simulink model "QuadRotorPlant"  (R2014b)
settings: Solver=ode23t  StartTime=0.0  StopTime=15  RelTol=1e-3
undefined symbols (not defined in the file): Ap, getArbitraryAngle, getArbitraryAxis, kt, L, Pitch_0, rho, Roll_0, Rp, X, Y, Z, zInit
libraries: sm_lib x125, fl_lib x106, nesl_utility x49, elec_lib x12, aerolibtransform2 x4, aerolibconvert2 x2
(part 1 of 4)
settings Model: Creator=ppreethi  LastModifiedBy=syoon
settings DataIOCC: SaveOutput=off  SaveTime=off
settings DebuggingCC: UnderspecifiedInitializationDetection=Classic  MergeDetectMultiDrivingBlocksExec=none  StateNameClashWarn=warning
settings SimscapeCC: SelectedTab=SimMechanics2G

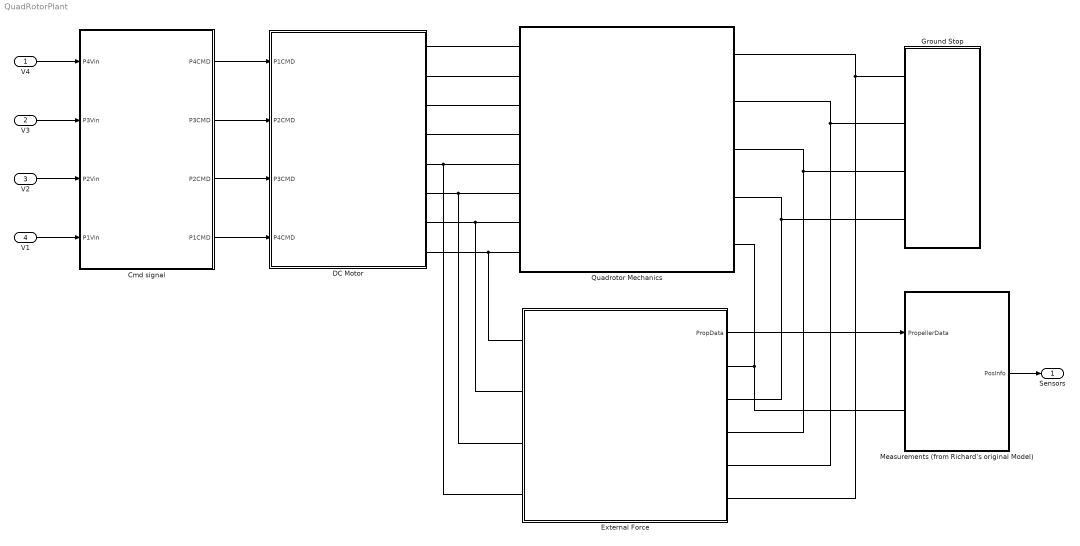
== system QuadRotorPlant ==
  V4 : Inport  OutDataTypeStr=double  PortDimensions=1  SampleTime=[0.01,0]
  V3 : Inport  Port=2  OutDataTypeStr=double  PortDimensions=1  SampleTime=[0.01,0]
  V2 : Inport  Port=3  OutDataTypeStr=double  PortDimensions=1  SampleTime=[0.01,0]
  V1 : Inport  Port=4  OutDataTypeStr=double  PortDimensions=1  SampleTime=[0.01,0]
  Cmd signal : Subsystem
  DC Motor : Subsystem
      mask Display: image(imread('motor.jpg'))
  External Force : Subsystem
  Ground Stop : Subsystem  mask{Roll0=Roll_0, Pitch0=Pitch_0, Yaw0=0, Damp=0.7, Spring=1e2, Length=-0.083057999999999979068, GRoll=0, GPitch=0, Alt=0}
      mask prompts: Roll0 "Init Roll"; Pitch0 "Init Pitch"; Yaw0 "Init Yaw"; Damp "Damping"; Spring "Spring Constant"; Length "Distance from Center to Motor"; GRoll "Ground Roll"; GPitch "Ground Pitch"; Alt "Initial Altitude"
      mask init:
      | blk = gcb;
      | if Alt<0
      |     Alt = 0;
      |     set_param(blk,'Alt','0')
      |     warning('Cannot Initialize Below Zero Altitude');
      | end
  Measurements (from Richard's original Model) : Subsystem
  Quadrotor Mechanics : Subsystem
  Sensors : Outport  OutDataTypeStr=Bus: VehicleStates  PortDimensions=1  SampleTime=0  BusOutputAsStruct=on
  wires:
  Cmd signal/1(P4CMD) -> DC Motor/1(P1CMD)
  Cmd signal/2(P3CMD) -> DC Motor/2(P2CMD)
  Cmd signal/3(P2CMD) -> DC Motor/3(P3CMD)
  Cmd signal/4(P1CMD) -> DC Motor/4(P4CMD)
  Measurements (from Richard's original Model)/1(PosInfo) -> Sensors/1
  V2/1 -> Cmd signal/3(P2Vin)
  V3/1 -> Cmd signal/2(P3Vin)
  V1/1 -> Cmd signal/4(P1Vin)
  V4/1 -> Cmd signal/1(P4Vin)
  External Force/1(PropData) -> Measurements (from Richard's original Model)/1(PropellerData)
  connections:
  Quadrotor Mechanics/LConn8 -- External Force/LConn1 -- DC Motor/RConn8
  External Force/LConn2 -- Quadrotor Mechanics/LConn7 -- DC Motor/RConn7
  External Force/LConn4 -- DC Motor/RConn5 -- Quadrotor Mechanics/LConn5
  Ground Stop/RConn1 -- External Force/RConn5 -- Quadrotor Mechanics/RConn1
  Ground Stop/RConn3 -- External Force/RConn3 -- Quadrotor Mechanics/RConn3
  Ground Stop/RConn2 -- External Force/RConn4 -- Quadrotor Mechanics/RConn2
  Ground Stop/RConn4 -- External Force/RConn2 -- Quadrotor Mechanics/RConn4
  External Force/RConn1 -- Measurements (from Richard's original Model)/LConn1 -- Quadrotor Mechanics/RConn5
  Quadrotor Mechanics/LConn6 -- External Force/LConn3 -- DC Motor/RConn6
  DC Motor/RConn4 -- Quadrotor Mechanics/LConn4
  DC Motor/RConn3 -- Quadrotor Mechanics/LConn3
  DC Motor/RConn2 -- Quadrotor Mechanics/LConn2
  DC Motor/RConn1 -- Quadrotor Mechanics/LConn1

== system QuadRotorPlant/Cmd signal ==
  P4Vin : Inport
  P3Vin : Inport  Port=2
  P2Vin : Inport  Port=3
  P1Vin : Inport  Port=4
  Bus Creator{1..4} (4 alike) : BusCreator  Inputs=2
  CMD : Subsystem
  CMD1 : Subsystem
  CMD2 : Subsystem
  CMD3 : Subsystem
  P4CMD : Outport
  P3CMD : Outport  Port=2
  P2CMD : Outport  Port=3
  P1CMD : Outport  Port=4
  wires:
  CMD3/2(REV) -> Bus Creator3/2  "rev"
  CMD3/1(Duty) -> Bus Creator3/1  "duty"
  CMD2/2(REV) -> Bus Creator2/2  "rev"
  CMD2/1(Duty) -> Bus Creator2/1  "duty"
  CMD1/2(REV) -> Bus Creator1/2  "rev"
  CMD1/1(Duty) -> Bus Creator1/1  "duty"
  Bus Creator1/1 -> P3CMD/1  "P2CMD"
  Bus Creator3/1 -> P1CMD/1  "P4CMD"
  Bus Creator2/1 -> P2CMD/1  "P3CMD"
  CMD/2(REV) -> Bus Creator4/2  "rev"
  CMD/1(Duty) -> Bus Creator4/1  "duty"
  Bus Creator4/1 -> P4CMD/1  "P1CMD"
  P3Vin/1 -> CMD1/1(Vcmd)
  P1Vin/1 -> CMD3/1(Vcmd)
  P2Vin/1 -> CMD2/1(Vcmd)
  P4Vin/1 -> CMD/1(Vcmd)

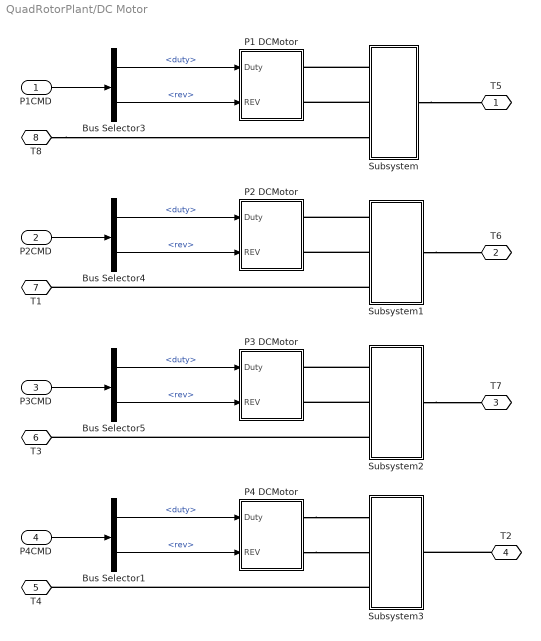
== system QuadRotorPlant/DC Motor ==
  P1CMD : Inport
  P2CMD : Inport  Port=2
  P3CMD : Inport  Port=3
  P4CMD : Inport  Port=4
  Bus Selector{1,3..5} (4 alike) : BusSelector  OutputSignals=duty,rev
  P1 DCMotor : Subsystem
      mask Display: image(imread('motor.jpg'))
  P2 DCMotor : Subsystem
      mask Display: image(imread('motor.jpg'))
  P3 DCMotor : Subsystem
      mask Display: image(imread('motor.jpg'))
  P4 DCMotor : Subsystem
      mask Display: image(imread('motor.jpg'))
  Subsystem : Subsystem
  Subsystem1 : Subsystem
  Subsystem2 : Subsystem
  Subsystem3 : Subsystem
  T5 : PMIOPort  Port=1  Side=Right
  T6 : PMIOPort  Port=2  Side=Right
  T7 : PMIOPort  Port=3  Side=Right
  T2 : PMIOPort  Port=4  Side=Right
  T4 : PMIOPort  Port=5  Side=Right
  T3 : PMIOPort  Port=6  Side=Right
  T1 : PMIOPort  Port=7  Side=Right
  T8 : PMIOPort  Port=8  Side=Right
  wires:
  Bus Selector1/1 -> P4 DCMotor/1(Duty)  "<duty>"
  Bus Selector1/2 -> P4 DCMotor/2(REV)  "<rev>"
  Bus Selector5/1 -> P3 DCMotor/1(Duty)  "<duty>"
  Bus Selector5/2 -> P3 DCMotor/2(REV)  "<rev>"
  Bus Selector4/1 -> P2 DCMotor/1(Duty)  "<duty>"
  Bus Selector4/2 -> P2 DCMotor/2(REV)  "<rev>"
  P2CMD/1 -> Bus Selector4/1
  P4CMD/1 -> Bus Selector1/1
  P3CMD/1 -> Bus Selector5/1
  P1CMD/1 -> Bus Selector3/1
  Bus Selector3/1 -> P1 DCMotor/1(Duty)  "<duty>"
  Bus Selector3/2 -> P1 DCMotor/2(REV)  "<rev>"
  connections:
  T8/RConn1 -- Subsystem/LConn3
  Subsystem1/LConn3 -- T1/RConn1
  Subsystem2/LConn3 -- T3/RConn1
  Subsystem3/LConn3 -- T4/RConn1
  T2/RConn1 -- Subsystem3/RConn1
  Subsystem2/RConn1 -- T7/RConn1
  Subsystem1/RConn1 -- T6/RConn1
  Subsystem/RConn1 -- T5/RConn1
  P4 DCMotor/RConn2 -- Subsystem3/LConn2
  P4 DCMotor/RConn1 -- Subsystem3/LConn1
  Subsystem2/LConn1 -- P3 DCMotor/RConn1
  Subsystem2/LConn2 -- P3 DCMotor/RConn2
  Subsystem1/LConn1 -- P2 DCMotor/RConn1
  Subsystem1/LConn2 -- P2 DCMotor/RConn2
  Subsystem/LConn2 -- P1 DCMotor/RConn2
  Subsystem/LConn1 -- P1 DCMotor/RConn1

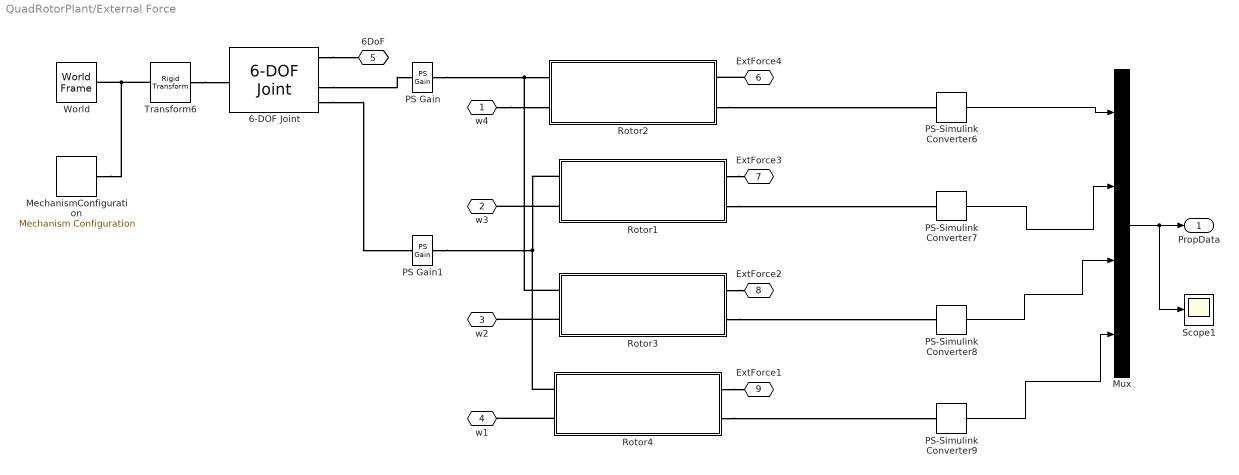
== system QuadRotorPlant/External Force ==
  6-DOF Joint : sm_lib/Joints/6-DOF Joint  SenseConstraintForce=off  SenseConstraintForceX=off  SenseConstraintForceY=off  SenseConstraintForceZ=off  SenseConstraintTorque=off  SenseConstraintTorqueX=off  SenseConstraintTorqueY=off  SenseConstraintTorqueZ=off  SenseTotalForce=off  SenseTotalForceX=off  SenseTotalForceY=off  SenseTotalForceZ=off  SenseTotalTorque=off  SenseTotalTorqueX=off  SenseTotalTorqueY=off  SenseTotalTorqueZ=off  CompositeWrenchDir=FollowerOnBase  CompositeWrenchFrame=BaseFrame  PxEquilibriumPosition=0  PxEquilibriumPositionUnits=m  PxSpringStiffness=0  PxSpringStiffnessUnits=N/m  PxDampingCoefficient=0  PxDampingCoefficientUnits=N/(m/s)  PxTorqueActuationMode=NoTorque  PxMotionActuationMode=ComputedMotion  PxSensePosition=off  PxSenseVelocity=off  PxSenseAcceleration=off  PxSenseTorqueForce=off  PxPositionTargetValue=0  PxPositionTargetValueUnits=m  PxPositionTargetSpecify=off  PxPositionTargetPriority=High  PxVelocityTargetValue=0  PxVelocityTargetValueUnits=m/s  PxVelocityTargetSpecify=off  PxVelocityTargetPriority=High  PyEquilibriumPosition=0  PyEquilibriumPositionUnits=m  PySpringStiffness=0  PySpringStiffnessUnits=N/m  PyDampingCoefficient=0  PyDampingCoefficientUnits=N/(m/s)  PyTorqueActuationMode=NoTorque  PyMotionActuationMode=ComputedMotion  PySensePosition=off  PySenseVelocity=off  PySenseAcceleration=off  PySenseTorqueForce=off  PyPositionTargetValue=0  PyPositionTargetValueUnits=m  PyPositionTargetSpecify=off  PyPositionTargetPriority=High  PyVelocityTargetValue=0  PyVelocityTargetValueUnits=m/s  PyVelocityTargetSpecify=off  PyVelocityTargetPriority=High  PzEquilibriumPosition=0  PzEquilibriumPositionUnits=m  PzSpringStiffness=0  PzSpringStiffnessUnits=N/m  PzDampingCoefficient=0  PzDampingCoefficientUnits=N/(m/s)  PzTorqueActuationMode=NoTorque  PzMotionActuationMode=ComputedMotion  PzSensePosition=off  PzSenseVelocity=on  PzSenseAcceleration=off  PzSenseTorqueForce=off  PzPositionTargetValue=0  PzPositionTargetValueUnits=m  PzPositionTargetSpecify=off  PzPositionTargetPriority=High  PzVelocityTargetValue=0  PzVelocityTargetValueUnits=m/s  PzVelocityTargetSpecify=off  PzVelocityTargetPriority=High  SphDefPosRotationMethod=None  SphDefPosRotationAngleUnits=deg  SphDefPosRotationStandardAxis=+Z  SphDefPosRotationAngle=0  SphDefPosRotationArbitraryAxis=[0 0 1]  SphDefPosFollAlignAxisA=+X  SphDefPosBaseAlignAxisA=+Y  SphDefPosFollAlignAxisB=+Y  SphDefPosBaseAlignAxisB=+Z  SphDefPosRotationMatrix=[1 0 0; 0 1 0; 0 0 1]  SphEqPosRotationMethod=None  SphEqPosRotationAngleUnits=deg  SphEqPosRotationStandardAxis=+Z  SphEqPosRotationAngle=0  SphEqPosRotationArbitraryAxis=[0 0 1]  SphEqPosFollAlignAxisA=+X  SphEqPosBaseAlignAxisA=+Y  SphEqPosFollAlignAxisB=+Y  SphEqPosBaseAlignAxisB=+Z  SphEqPosRotationMatrix=[1 0 0; 0 1 0; 0 0 1]  SphSpringStiffness=0  SphSpringStiffnessUnits=N*m/deg  SphDampingCoefficient=0  SphDampingCoefficientUnits=N*m/(deg/s)  SphActuateTorqueX=off  SphActuateTorqueY=off  SphActuateTorqueZ=off  SphActuateTorque=off  SphTorqueActuationMode=NoTorque  SphMotionActuationMode=ComputedMotion  SphActuationFrame=BaseFrame  SphSensePosition=off  SphSenseVelocityX=on  SphSenseVelocityY=on  SphSenseVelocityZ=off  SphSenseVelocity=off  SphSenseAccelerationX=off  SphSenseAccelerationY=off  SphSenseAccelerationZ=off  SphSenseAcceleration=off  SphSenseTorqueX=off  SphSenseTorqueY=off  SphSenseTorqueZ=off  SphSenseTorqueForce=off  SphSensingFrame=BaseFrame  SphPositionTargetRotationMethod=None  SphPositionTargetRotationAngleUnits=deg  SphPositionTargetRotationStandardAxis=+Z  SphPositionTargetRotationAngle=0  SphPositionTargetRotationArbitraryAxis=[0 0 1]  SphPositionTargetFollAlignAxisA=+X  SphPositionTargetBaseAlignAxisA=+Y  SphPositionTargetFollAlignAxisB=+Y  SphPositionTargetBaseAlignAxisB=+Z  SphPositionTargetRotationMatrix=[1 0 0; 0 1 0; 0 0 1]  SphPositionTargetSpecify=off  SphPositionTargetPriority=High  SphVelocityTargetValue=[0 0 0]  SphVelocityTargetValueUnits=deg/s  SphVelocityTargetSpecify=off  SphVelocityTargetPriority=High  SphVelocityTargetInFollowerFrame=on  BlockFunction=simmechanics.library.joints.sixdof_joint
  MechanismConfiguration : sm_lib/Utilities/Mechanism Configuration  UniformGravity=Constant  GravityVector=[0 0 9.81]  GravityUnits=m/s^2  LinearizationDelta=0.001  BlockFunction=simmechanics.library.utilities.mechanism_configuration
  Mux : Mux
  PS Gain : fl_lib/Physical Signals/Functions/PS Gain  gain=pi/180
  PS Gain1 : fl_lib/Physical Signals/Functions/PS Gain  gain=pi/180
  PS-Simulink Converter{6..9} (4 alike) : nesl_utility/PS-Simulink Converter  PhysicalDomain=network_engine_domain  SubClassName=ps_output  LeftPortType=input  RightPortType=output  PseudoPeriodic=off  Frequencies=[]  Unit=1  AffineConversion=off
  Rotor1 : Subsystem
  Rotor2 : Subsystem
  Rotor3 : Subsystem
  Rotor4 : Subsystem
  Scope1 : Scope
      settings: TimeRange=5  YMin=-0.025  YMax=0.25  SaveName=ScopeData11
  Transform6 : sm_lib/Frames and Transforms/Rigid Transform  TranslationMethod=None  TranslationLengthUnit=m  TranslationStandardAxis=+Z  TranslationStandardOffset=0  TranslationCartesianOffset=[0 0 0]  TranslationROffset=0  TranslationROffsetUnits=m  TranslationZOffset=0  TranslationZOffsetUnits=m  TranslationThetaOffset=0  TranslationThetaOffsetUnits=deg  RotationMethod=StandardAxis  RotationAngleUnits=deg  RotationStandardAxis=+X  RotationAngle=180  RotationArbitraryAxis=[0 0 1]  FollAlignAxisA=+X  BaseAlignAxisA=+Y  FollAlignAxisB=+Y  BaseAlignAxisB=+Z  RotationMatrix=[1 0 0; 0 1 0; 0 0 1]  BlockFunction=simmechanics.library.frames_transforms.rigid_transform
  World : sm_lib/Frames and Transforms/World Frame  BlockFunction=simmechanics.library.frames_transforms.world_frame
  w4 : PMIOPort  Port=1  Side=Left
  w3 : PMIOPort  Port=2  Side=Left
  w2 : PMIOPort  Port=3  Side=Left
  w1 : PMIOPort  Port=4  Side=Left
  6DoF : PMIOPort  Port=5  Side=Right
  ExtForce4 : PMIOPort  Port=6  Side=Right
  ExtForce3 : PMIOPort  Port=7  Side=Right
  ExtForce2 : PMIOPort  Port=8  Side=Right
  ExtForce1 : PMIOPort  Port=9  Side=Right
  PropData : Outport
  wires:
  Mux/1 -> PropData/1, Scope1/1
  PS-Simulink Converter6/1 -> Mux/1
  PS-Simulink Converter7/1 -> Mux/2
  PS-Simulink Converter8/1 -> Mux/3
  PS-Simulink Converter9/1 -> Mux/4
  connections:
  6-DOF Joint/RConn3 -- PS Gain/LConn1
  6-DOF Joint/RConn4 -- PS Gain1/LConn1
  MechanismConfiguration/RConn1 -- World/RConn1 -- Transform6/LConn1
  Transform6/RConn1 -- 6-DOF Joint/LConn1
  6-DOF Joint/RConn1 -- 6DoF/RConn1
  Rotor4/LConn2 -- w1/RConn1
  Rotor3/LConn2 -- w2/RConn1
  w4/RConn1 -- Rotor2/LConn2
  ExtForce4/RConn1 -- Rotor2/RConn1
  Rotor1/RConn1 -- ExtForce3/RConn1
  Rotor2/RConn2 -- PS-Simulink Converter6/LConn1
  PS Gain/RConn1 -- Rotor3/LConn1 -- Rotor2/LConn1
  Rotor3/RConn1 -- ExtForce2/RConn1
  Rotor1/LConn1 -- Rotor4/LConn1 -- PS Gain1/RConn1
  Rotor1/RConn2 -- PS-Simulink Converter7/LConn1
  Rotor1/LConn2 -- w3/RConn1
  Rotor3/RConn2 -- PS-Simulink Converter8/LConn1
  Rotor4/RConn2 -- PS-Simulink Converter9/LConn1
  Rotor4/RConn1 -- ExtForce1/RConn1

== system QuadRotorPlant/Ground Stop ==
  FloorStop1 : Subsystem
  FloorStop2 : Subsystem
  FloorStop3 : Subsystem
  FloorStop4 : Subsystem
  Ground : sm_lib/Body Elements/Solid  InertiaType=CalculateFromGeometry  Mass=1  MassUnits=kg  CenterOfMass=[0 0 0]  CenterOfMassUnits=m  MomentsOfInertia=[1 1 1]  MomentsOfInertiaUnits=kg*m^2  ProductsOfInertia=[0 0 0]  ProductsOfInertiaUnits=kg*m^2  DensityBased=on  Density=2000  DensityUnits=kg/(m^3)  GraphicType=FromGeometry  MarkerShape=Sphere  MarkerSize=10  MarkerSizeUnits=m  GraphicVisPropType=SimpleVisualProperties  GraphicDiffuseColor=[0.0 0.0 0.2]  GraphicSpecularColor=[0.5 0.5 0.5 1.0]  GraphicAmbientColor=[0.15 0.15 0.15 1.0]  GraphicEmissiveColor=[0.0 0.0 0.0 1.0]  GraphicShininess=75  GraphicOpacity=1.0  GeometryShape=Brick  RectangleSize=[1 1]  RectangleSizeUnits=m  BrickDimensions=[1 1 0.01]  BrickDimensionUnits=m  CylinderRadius=1  CylinderRadiusUnits=m  CylinderLength=1  CylinderLengthUnits=m  SphereRadius=1  SphereRadiusUnits=m  EllipsoidRadii=[1 1 1]  EllipsoidRadiiUnits=m  ExtrusionCrossSection=[1 1; -1 1; -1 -1; 1 -1]  ExtrusionCrossSectionUnits=m  ExtrusionLength=1  ExtrusionLengthUnits=m  PolygonNumSides=3  PolygonOuterRadius=1  PolygonOuterRadiusUnits=m  ExtGeomFileType=STL  ExtGeomFileUnits=m  RevolutionCrossSection=[1 1; 1 -1; 2 -1; 2 1]  RevolutionCrossSectionUnits=m  RevolutionExtent=Full  RevolutionAngle=180  RevolutionAngleUnits=deg  BlockFunction=simmechanics.library.body_elements.solid
  Transform1 : sm_lib/Frames and Transforms/Rigid Transform  TranslationMethod=None  TranslationLengthUnit=m  TranslationStandardAxis=+Z  TranslationStandardOffset=0  TranslationCartesianOffset=[0 0 -Alt-0.038]  TranslationROffset=0  TranslationROffsetUnits=m  TranslationZOffset=0  TranslationZOffsetUnits=m  TranslationThetaOffset=0  TranslationThetaOffsetUnits=deg  RotationMethod=ArbitraryAxis  RotationAngleUnits=deg  RotationStandardAxis=+X  RotationAngle=-getArbitraryAngle(GPitch,GRoll,Yaw0)  RotationArbitraryAxis=getArbitraryAxis(GPitch,GRoll,Yaw0);  FollAlignAxisA=-Z  BaseAlignAxisA=+Y  FollAlignAxisB=-Y  BaseAlignAxisB=+X  RotationMatrix=[1 0 0; 0 1 0; 0 0 1]  BlockFunction=simmechanics.library.frames_transforms.rigid_transform
  Transform2 : sm_lib/Frames and Transforms/Rigid Transform  TranslationMethod=Cartesian  TranslationLengthUnit=m  TranslationStandardAxis=+Z  TranslationStandardOffset=0  TranslationCartesianOffset=[0 0 -Alt-0.038]  TranslationROffset=0  TranslationROffsetUnits=m  TranslationZOffset=0  TranslationZOffsetUnits=m  TranslationThetaOffset=0  TranslationThetaOffsetUnits=deg  RotationMethod=StandardAxis  RotationAngleUnits=deg  RotationStandardAxis=+X  RotationAngle=180  RotationArbitraryAxis=getArbitraryAxis(GRoll,GPitch,0);  FollAlignAxisA=-Z  BaseAlignAxisA=+Y  FollAlignAxisB=-Y  BaseAlignAxisB=+X  RotationMatrix=[1 0 0; 0 1 0; 0 0 1]  BlockFunction=simmechanics.library.frames_transforms.rigid_transform
  Transform6 : sm_lib/Frames and Transforms/Rigid Transform  TranslationMethod=None  TranslationLengthUnit=m  TranslationStandardAxis=+Z  TranslationStandardOffset=0  TranslationCartesianOffset=[0 0 0]  TranslationROffset=0  TranslationROffsetUnits=m  TranslationZOffset=0  TranslationZOffsetUnits=m  TranslationThetaOffset=0  TranslationThetaOffsetUnits=deg  RotationMethod=StandardAxis  RotationAngleUnits=deg  RotationStandardAxis=+X  RotationAngle=180  RotationArbitraryAxis=[0 0 1]  FollAlignAxisA=+X  BaseAlignAxisA=+Y  FollAlignAxisB=+Y  BaseAlignAxisB=+Z  RotationMatrix=[1 0 0; 0 1 0; 0 0 1]  BlockFunction=simmechanics.library.frames_transforms.rigid_transform
  World1 : sm_lib/Frames and Transforms/World Frame  BlockFunction=simmechanics.library.frames_transforms.world_frame
  Conn1 : PMIOPort  Port=1  Side=Right
  Conn2 : PMIOPort  Port=2  Side=Right
  Conn3 : PMIOPort  Port=3  Side=Right
  Conn4 : PMIOPort  Port=4  Side=Right
  connections:
  Transform6/LConn1 -- World1/RConn1
  Transform1/RConn1 -- Transform2/LConn1
  Transform1/LConn1 -- Ground/RConn1
  FloorStop1/LConn1 -- FloorStop4/LConn1 -- FloorStop2/LConn1 -- Transform2/RConn1 -- Transform6/RConn1 -- FloorStop3/LConn1
  Conn4/RConn1 -- FloorStop3/RConn1
  Conn2/RConn1 -- FloorStop2/RConn1
  Conn3/RConn1 -- FloorStop1/RConn1
  FloorStop4/RConn1 -- Conn1/RConn1

== system QuadRotorPlant/Measurements (from Richard's original Model) ==
  PropellerData : Inport
  Aerodynamic Drag : Subsystem
  6dof : PMIOPort  Port=1  Side=Left
  PosInfo : Outport  OutDataTypeStr=Bus: VehicleStates
  wires:
  PropellerData/1 -> Aerodynamic Drag/1(PropData)
  Aerodynamic Drag/1(posInfo) -> PosInfo/1
  connections:
  Aerodynamic Drag/LConn1 -- 6dof/RConn1

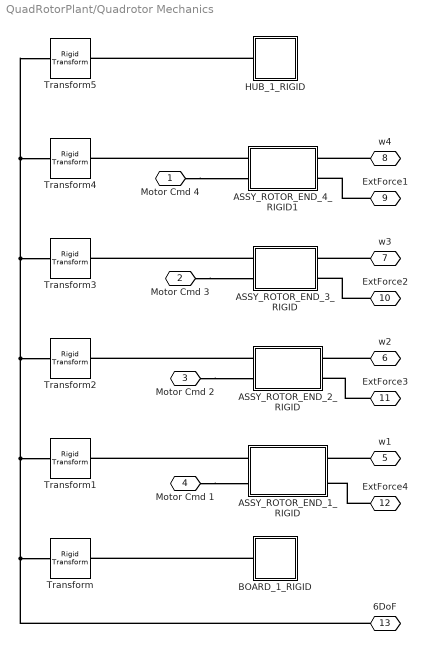
== system QuadRotorPlant/Quadrotor Mechanics ==
  ASSY_ROTOR_END_1_RIGID : Subsystem
  ASSY_ROTOR_END_2_RIGID : Subsystem
  ASSY_ROTOR_END_3_RIGID : Subsystem
  ASSY_ROTOR_END_4_RIGID1 : Subsystem
  BOARD_1_RIGID : Subsystem
  HUB_1_RIGID : Subsystem
  Transform : sm_lib/Frames and Transforms/Rigid Transform  TranslationMethod=Cartesian  TranslationLengthUnit=in  TranslationStandardAxis=+Z  TranslationStandardOffset=0  TranslationCartesianOffset=[0 0 0.27699999999999997]  TranslationROffset=0  TranslationROffsetUnits=m  TranslationZOffset=0  TranslationZOffsetUnits=m  TranslationThetaOffset=0  TranslationThetaOffsetUnits=deg  RotationMethod=ArbitraryAxis  RotationAngleUnits=rad  RotationStandardAxis=+Z  RotationAngle=2.3561943620144121  RotationArbitraryAxis=[-0 -0 -0.99999999999999989]  FollAlignAxisA=+X  BaseAlignAxisA=+Y  FollAlignAxisB=+Y  BaseAlignAxisB=+Z  RotationMatrix=[1 0 0; 0 1 0; 0 0 1]  BlockFunction=simmechanics.library.frames_transforms.rigid_transform
  Transform1 : sm_lib/Frames and Transforms/Rigid Transform  TranslationMethod=Cartesian  TranslationLengthUnit=in  TranslationStandardAxis=+Z  TranslationStandardOffset=0  TranslationCartesianOffset=[0.085999999999999979 -5.5118110236220464e-05 5.5118110236220464e-05]  TranslationROffset=0  TranslationROffsetUnits=m  TranslationZOffset=0  TranslationZOffsetUnits=m  TranslationThetaOffset=0  TranslationThetaOffsetUnits=deg  RotationMethod=None  RotationAngleUnits=deg  RotationStandardAxis=+Z  RotationAngle=0  RotationArbitraryAxis=[0 0 1]  FollAlignAxisA=+X  BaseAlignAxisA=+Y  FollAlignAxisB=+Y  BaseAlignAxisB=+Z  RotationMatrix=[1 0 0; 0 1 0; 0 0 1]  BlockFunction=simmechanics.library.frames_transforms.rigid_transform
  Transform2 : sm_lib/Frames and Transforms/Rigid Transform  TranslationMethod=Cartesian  TranslationLengthUnit=in  TranslationStandardAxis=+Z  TranslationStandardOffset=0  TranslationCartesianOffset=[-5.5118110236220464e-05 -0.085999999999999979 5.5118110236220464e-05]  TranslationROffset=0  TranslationROffsetUnits=m  TranslationZOffset=0  TranslationZOffsetUnits=m  TranslationThetaOffset=0  TranslationThetaOffsetUnits=deg  RotationMethod=ArbitraryAxis  RotationAngleUnits=rad  RotationStandardAxis=+Z  RotationAngle=1.5707963267948968  RotationArbitraryAxis=[-0 -0 -1]  FollAlignAxisA=+X  BaseAlignAxisA=+Y  FollAlignAxisB=+Y  BaseAlignAxisB=+Z  RotationMatrix=[1 0 0; 0 1 0; 0 0 1]  BlockFunction=simmechanics.library.frames_transforms.rigid_transform
  Transform3 : sm_lib/Frames and Transforms/Rigid Transform  TranslationMethod=Cartesian  TranslationLengthUnit=in  TranslationStandardAxis=+Z  TranslationStandardOffset=0  TranslationCartesianOffset=[-0.085999999999999979 5.5118110236220464e-05 5.5118110236220464e-05]  TranslationROffset=0  TranslationROffsetUnits=m  TranslationZOffset=0  TranslationZOffsetUnits=m  TranslationThetaOffset=0  TranslationThetaOffsetUnits=deg  RotationMethod=ArbitraryAxis  RotationAngleUnits=rad  RotationStandardAxis=+Z  RotationAngle=3.1415926535897931  RotationArbitraryAxis=[0 0 1]  FollAlignAxisA=+X  BaseAlignAxisA=+Y  FollAlignAxisB=+Y  BaseAlignAxisB=+Z  RotationMatrix=[1 0 0; 0 1 0; 0 0 1]  BlockFunction=simmechanics.library.frames_transforms.rigid_transform
  Transform4 : sm_lib/Frames and Transforms/Rigid Transform  TranslationMethod=Cartesian  TranslationLengthUnit=in  TranslationStandardAxis=+Z  TranslationStandardOffset=0  TranslationCartesianOffset=[5.5118110236220464e-05 0.085999999999999979 5.5118110236220464e-05]  TranslationROffset=0  TranslationROffsetUnits=m  TranslationZOffset=0  TranslationZOffsetUnits=m  TranslationThetaOffset=0  TranslationThetaOffsetUnits=deg  RotationMethod=ArbitraryAxis  RotationAngleUnits=rad  RotationStandardAxis=+Z  RotationAngle=1.5707963267948968  RotationArbitraryAxis=[0 0 1]  FollAlignAxisA=+X  BaseAlignAxisA=+Y  FollAlignAxisB=+Y  BaseAlignAxisB=+Z  RotationMatrix=[1 0 0; 0 1 0; 0 0 1]  BlockFunction=simmechanics.library.frames_transforms.rigid_transform
  Transform5 : sm_lib/Frames and Transforms/Rigid Transform  TranslationMethod=None  TranslationLengthUnit=m  TranslationStandardAxis=+Z  TranslationStandardOffset=0  TranslationCartesianOffset=[0 0 0]  TranslationROffset=0  TranslationROffsetUnits=m  TranslationZOffset=0  TranslationZOffsetUnits=m  TranslationThetaOffset=0  TranslationThetaOffsetUnits=deg  RotationMethod=None  RotationAngleUnits=deg  RotationStandardAxis=+Z  RotationAngle=0  RotationArbitraryAxis=[0 0 1]  FollAlignAxisA=+X  BaseAlignAxisA=+Y  FollAlignAxisB=+Y  BaseAlignAxisB=+Z  RotationMatrix=[1 0 0; 0 1 0; 0 0 1]  BlockFunction=simmechanics.library.frames_transforms.rigid_transform
  Motor Cmd 4 : PMIOPort  Port=1  Side=Left
  Motor Cmd 3 : PMIOPort  Port=2  Side=Left
  Motor Cmd 2 : PMIOPort  Port=3  Side=Left
  Motor Cmd 1 : PMIOPort  Port=4  Side=Left
  w1 : PMIOPort  Port=5  Side=Left
  w2 : PMIOPort  Port=6  Side=Left
  w3 : PMIOPort  Port=7  Side=Left
  w4 : PMIOPort  Port=8  Side=Left
  ExtForce1 : PMIOPort  Port=9  Side=Right
  ExtForce2 : PMIOPort  Port=10  Side=Right
  ExtForce3 : PMIOPort  Port=11  Side=Right
  ExtForce4 : PMIOPort  Port=12  Side=Right
  6DoF : PMIOPort  Port=13  Side=Right
  connections:
  ASSY_ROTOR_END_4_RIGID1/LConn1 -- Transform4/RConn1
  ASSY_ROTOR_END_2_RIGID/LConn1 -- Transform2/RConn1
  6DoF/RConn1 -- Transform1/LConn1 -- Transform2/LConn1 -- Transform3/LConn1 -- Transform5/LConn1 -- Transform4/LConn1 -- Transform/LConn1
  ASSY_ROTOR_END_1_RIGID/LConn1 -- Transform1/RConn1
  BOARD_1_RIGID/LConn1 -- Transform/RConn1
  ASSY_ROTOR_END_3_RIGID/LConn1 -- Transform3/RConn1
  HUB_1_RIGID/LConn1 -- Transform5/RConn1
  Motor Cmd 1/RConn1 -- ASSY_ROTOR_END_1_RIGID/LConn2
  w3/RConn1 -- ASSY_ROTOR_END_3_RIGID/RConn1
  Motor Cmd 2/RConn1 -- ASSY_ROTOR_END_2_RIGID/LConn2
  w2/RConn1 -- ASSY_ROTOR_END_2_RIGID/RConn1
  ExtForce3/RConn1 -- ASSY_ROTOR_END_2_RIGID/RConn2
  ExtForce1/RConn1 -- ASSY_ROTOR_END_4_RIGID1/RConn2
  Motor Cmd 4/RConn1 -- ASSY_ROTOR_END_4_RIGID1/LConn2
  w4/RConn1 -- ASSY_ROTOR_END_4_RIGID1/RConn1
  Motor Cmd 3/RConn1 -- ASSY_ROTOR_END_3_RIGID/LConn2
  w1/RConn1 -- ASSY_ROTOR_END_1_RIGID/RConn1
  ExtForce4/RConn1 -- ASSY_ROTOR_END_1_RIGID/RConn2
  ExtForce2/RConn1 -- ASSY_ROTOR_END_3_RIGID/RConn2

== system QuadRotorPlant/Cmd signal/CMD ==
  Vcmd : Inport
  Abs : Abs
  Fcn : Fcn  Expr=u(1)>0
  Gain : Gain  Gain=4
  "[0...4]" : Saturate  UpperLimit=4  LowerLimit=0
  Duty : Outport
  REV : Outport  Port=2
  wires:
  Vcmd/1 -> Fcn/1, Abs/1
  Abs/1 -> "[0...4]"/1
  Fcn/1 -> Gain/1
  "[0...4]"/1 -> Duty/1
  Gain/1 -> REV/1

== system QuadRotorPlant/Cmd signal/CMD1 ==
  Vcmd : Inport
  Abs : Abs
  Fcn : Fcn  Expr=u(1)>0
  Gain : Gain  Gain=4
  "[0...4]" : Saturate  UpperLimit=4  LowerLimit=0
  Duty : Outport
  REV : Outport  Port=2
  wires:
  Gain/1 -> REV/1
  "[0...4]"/1 -> Duty/1
  Fcn/1 -> Gain/1
  Abs/1 -> "[0...4]"/1
  Vcmd/1 -> Abs/1, Fcn/1

== system QuadRotorPlant/Cmd signal/CMD2 ==
  Vcmd : Inport
  Abs : Abs
  Fcn : Fcn  Expr=u(1)>0
  Gain : Gain  Gain=4
  "[0...4]" : Saturate  UpperLimit=4  LowerLimit=0
  Duty : Outport
  REV : Outport  Port=2
  wires:
  Vcmd/1 -> Fcn/1, Abs/1
  Abs/1 -> "[0...4]"/1
  Fcn/1 -> Gain/1
  "[0...4]"/1 -> Duty/1
  Gain/1 -> REV/1

== system QuadRotorPlant/Cmd signal/CMD3 ==
  Vcmd : Inport
  Abs : Abs
  Fcn : Fcn  Expr=u(1)>0
  Gain : Gain  Gain=4
  "[0...4]" : Saturate  UpperLimit=4  LowerLimit=0
  Duty : Outport
  REV : Outport  Port=2
  wires:
  Gain/1 -> REV/1
  "[0...4]"/1 -> Duty/1
  Fcn/1 -> Gain/1
  Abs/1 -> "[0...4]"/1
  Vcmd/1 -> Abs/1, Fcn/1

== system QuadRotorPlant/DC Motor/P1 DCMotor ==
  Duty : Inport
  REV : Inport  Port=2
  DC Motor : elec_lib/Actuators & Drivers/Rotational Actuators/DC Motor  parameterization=3  Ra=3.9 Ohm  La=0.001 H  emf_or_torque=1  Kv=1/7000 V/rpm  Ki=6.876e-04 N*m/A  T_stall=2.4e-04 N*m  w_max=4*7000 rpm  w_rated=25000 rpm  P_rated=10 W  V_rated=4 V  J=2 g*cm^2  lam_param=1  lam=1e-06 N*m/(rad/s)  i_noload=0 A  V_i_noload=1.5 V  speed0=0 rpm  alpha=0.00393 1/K  Tmeas=25 C  thermal_mass=100 J/K  initial_temperature=25 C
  Electrical Reference2 : fl_lib/Electrical/Electrical Elements/Electrical Reference
  Mechanical Rotational Reference : fl_lib/Mechanical/Rotational Elements/Mechanical Rotational Reference
  Power Amplifier : Subsystem
  Solver Configuration : nesl_utility/Solver Configuration  PhysicalDomain=network_engine_domain  SubClassName=solver  LeftPortType=input  RightPortType=generic  Accelerate=off  Tones=[]  Harmonics=[]  SimulateNoise=off  Profile=off  UseLocalSampling=off  EnableSwitchedLinearOptims=on  FrequencyDomain=off  UseCCode=off  RelTol=0.001  AbsTol=1e-06  MinStep=1e-09  ToWorkspace=off  DoDC=off  ResidualTolerance=1e-09  UseLocalSolver=off  LocalSolverChoice=NE_BACKWARD_EULER_ADVANCER  LocalSolverSampleTime=0.001  DoFixedCost=off  MaxNonlinIter=3  MaxModeIter=2  LinearAlgebra=Sparse  DelaysMemoryBudget=1024  AutomaticFiltering=on  FilteringTimeConstant=0.001
  Shaft : PMIOPort  Tag=PMCPort  Port=1  Side=Right
  Housing : PMIOPort  Tag=PMCPort  Port=2  Side=Right
  wires:
  REV/1 -> Power Amplifier/2(REV)
  Duty/1 -> Power Amplifier/1(Duty)
  connections:
  DC Motor/RConn2 -- Housing/RConn1 -- Solver Configuration/RConn1 -- Mechanical Rotational Reference/LConn1
  Power Amplifier/RConn2 -- DC Motor/RConn1 -- Electrical Reference2/LConn1
  DC Motor/LConn2 -- Shaft/RConn1
  Power Amplifier/RConn1 -- DC Motor/LConn1

== system QuadRotorPlant/DC Motor/P2 DCMotor ==
  Duty : Inport
  REV : Inport  Port=2
  DC Motor : elec_lib/Actuators & Drivers/Rotational Actuators/DC Motor  parameterization=3  Ra=3.9 Ohm  La=0.001 H  emf_or_torque=1  Kv=1/7000 V/rpm  Ki=6.876e-04 N*m/A  T_stall=2.4e-04 N*m  w_max=4*7000 rpm  w_rated=25000 rpm  P_rated=10 W  V_rated=4 V  J=2 g*cm^2  lam_param=1  lam=1e-06 N*m/(rad/s)  i_noload=0 A  V_i_noload=1.5 V  speed0=0 rpm  alpha=0.00393 1/K  Tmeas=25 C  thermal_mass=100 J/K  initial_temperature=25 C
  Electrical Reference2 : fl_lib/Electrical/Electrical Elements/Electrical Reference
  Mechanical Rotational Reference : fl_lib/Mechanical/Rotational Elements/Mechanical Rotational Reference
  Power Amplifier : Subsystem
  Shaft : PMIOPort  Tag=PMCPort  Port=1  Side=Right
  Housing : PMIOPort  Tag=PMCPort  Port=2  Side=Right
  wires:
  Duty/1 -> Power Amplifier/1(Duty)
  REV/1 -> Power Amplifier/2(REV)
  connections:
  Power Amplifier/RConn1 -- DC Motor/LConn1
  DC Motor/LConn2 -- Shaft/RConn1
  Electrical Reference2/LConn1 -- DC Motor/RConn1 -- Power Amplifier/RConn2
  Mechanical Rotational Reference/LConn1 -- Housing/RConn1 -- DC Motor/RConn2

== system QuadRotorPlant/DC Motor/P3 DCMotor ==
  Duty : Inport
  REV : Inport  Port=2
  DC Motor : elec_lib/Actuators & Drivers/Rotational Actuators/DC Motor  parameterization=3  Ra=3.9 Ohm  La=0.001 H  emf_or_torque=1  Kv=1/7000 V/rpm  Ki=6.876e-04 N*m/A  T_stall=2.4e-04 N*m  w_max=4*7000 rpm  w_rated=25000 rpm  P_rated=10 W  V_rated=4 V  J=2 g*cm^2  lam_param=1  lam=1e-06 N*m/(rad/s)  i_noload=0 A  V_i_noload=1.5 V  speed0=0 rpm  alpha=0.00393 1/K  Tmeas=25 C  thermal_mass=100 J/K  initial_temperature=25 C
  Electrical Reference2 : fl_lib/Electrical/Electrical Elements/Electrical Reference
  Mechanical Rotational Reference : fl_lib/Mechanical/Rotational Elements/Mechanical Rotational Reference
  Power Amplifier : Subsystem
  Shaft : PMIOPort  Tag=PMCPort  Port=1  Side=Right
  Housing : PMIOPort  Tag=PMCPort  Port=2  Side=Right
  wires:
  REV/1 -> Power Amplifier/2(REV)
  Duty/1 -> Power Amplifier/1(Duty)
  connections:
  DC Motor/RConn2 -- Housing/RConn1 -- Mechanical Rotational Reference/LConn1
  Power Amplifier/RConn2 -- DC Motor/RConn1 -- Electrical Reference2/LConn1
  DC Motor/LConn2 -- Shaft/RConn1
  Power Amplifier/RConn1 -- DC Motor/LConn1

== system QuadRotorPlant/DC Motor/P4 DCMotor ==
  Duty : Inport
  REV : Inport  Port=2
  DC Motor : elec_lib/Actuators & Drivers/Rotational Actuators/DC Motor  parameterization=3  Ra=3.9 Ohm  La=0.001 H  emf_or_torque=1  Kv=1/7000 V/rpm  Ki=6.876e-04 N*m/A  T_stall=2.4e-04 N*m  w_max=4*7000 rpm  w_rated=25000 rpm  P_rated=10 W  V_rated=4 V  J=2 g*cm^2  lam_param=1  lam=1e-06 N*m/(rad/s)  i_noload=0 A  V_i_noload=1.5 V  speed0=0 rpm  alpha=0.00393 1/K  Tmeas=25 C  thermal_mass=100 J/K  initial_temperature=25 C
  Electrical Reference2 : fl_lib/Electrical/Electrical Elements/Electrical Reference
  Mechanical Rotational Reference : fl_lib/Mechanical/Rotational Elements/Mechanical Rotational Reference
  Power Amplifier : Subsystem
  Shaft : PMIOPort  Tag=PMCPort  Port=1  Side=Right
  Housing : PMIOPort  Tag=PMCPort  Port=2  Side=Right
  wires:
  Duty/1 -> Power Amplifier/1(Duty)
  REV/1 -> Power Amplifier/2(REV)
  connections:
  Power Amplifier/RConn1 -- DC Motor/LConn1
  DC Motor/LConn2 -- Shaft/RConn1
  Electrical Reference2/LConn1 -- DC Motor/RConn1 -- Power Amplifier/RConn2
  Mechanical Rotational Reference/LConn1 -- Housing/RConn1 -- DC Motor/RConn2

== system QuadRotorPlant/DC Motor/Subsystem ==
  Angular Velocity Source : fl_lib/Mechanical/Mechanical Sources/Ideal Angular Velocity Source
  Torque Sensor : fl_lib/Mechanical/Mechanical Sensors/Ideal Torque Sensor
  B : PMIOPort  Port=1  Side=Left
  F : PMIOPort  Port=2  Side=Left
  T2 : PMIOPort  Port=3  Side=Left
  T1 : PMIOPort  Port=4  Side=Right
  connections:
  Angular Velocity Source/LConn1 -- Torque Sensor/RConn1
  Angular Velocity Source/RConn2 -- B/RConn1
  Torque Sensor/LConn1 -- F/RConn1
  T2/RConn1 -- Angular Velocity Source/RConn1
  T1/RConn1 -- Torque Sensor/RConn2

== system QuadRotorPlant/DC Motor/Subsystem1 ==
  Angular Velocity Source : fl_lib/Mechanical/Mechanical Sources/Ideal Angular Velocity Source
  Torque Sensor : fl_lib/Mechanical/Mechanical Sensors/Ideal Torque Sensor
  B : PMIOPort  Port=1  Side=Left
  F : PMIOPort  Port=2  Side=Left
  T2 : PMIOPort  Port=3  Side=Left
  T1 : PMIOPort  Port=4  Side=Right
  connections:
  T1/RConn1 -- Torque Sensor/RConn2
  T2/RConn1 -- Angular Velocity Source/RConn1
  Torque Sensor/LConn1 -- F/RConn1
  Angular Velocity Source/RConn2 -- B/RConn1
  Angular Velocity Source/LConn1 -- Torque Sensor/RConn1

== system QuadRotorPlant/DC Motor/Subsystem2 ==
  Angular Velocity Source : fl_lib/Mechanical/Mechanical Sources/Ideal Angular Velocity Source
  Torque Sensor : fl_lib/Mechanical/Mechanical Sensors/Ideal Torque Sensor
  B : PMIOPort  Port=1  Side=Left
  F : PMIOPort  Port=2  Side=Left
  T2 : PMIOPort  Port=3  Side=Left
  T1 : PMIOPort  Port=4  Side=Right
  connections:
  Angular Velocity Source/LConn1 -- Torque Sensor/RConn1
  Angular Velocity Source/RConn2 -- B/RConn1
  Torque Sensor/LConn1 -- F/RConn1
  T2/RConn1 -- Angular Velocity Source/RConn1
  T1/RConn1 -- Torque Sensor/RConn2

== system QuadRotorPlant/DC Motor/Subsystem3 ==
  Angular Velocity Source : fl_lib/Mechanical/Mechanical Sources/Ideal Angular Velocity Source
  Torque Sensor : fl_lib/Mechanical/Mechanical Sensors/Ideal Torque Sensor
  B : PMIOPort  Port=1  Side=Left
  F : PMIOPort  Port=2  Side=Left
  T2 : PMIOPort  Port=3  Side=Left
  T1 : PMIOPort  Port=4  Side=Right
  connections:
  T1/RConn1 -- Torque Sensor/RConn2
  T2/RConn1 -- Angular Velocity Source/RConn1
  Torque Sensor/LConn1 -- F/RConn1
  Angular Velocity Source/RConn2 -- B/RConn1
  Angular Velocity Source/LConn1 -- Torque Sensor/RConn1

== system QuadRotorPlant/External Force/Rotor1 ==
  Display : Display
  External Force  and Torque1 : sm_lib/Forces and Torques/External Force and Torque  ForceResolutionFrame=AttachedFrame  EnableForceX=off  EnableForceY=off  EnableForceZ=on  EnableForce=off  TorqueResolutionFrame=AttachedFrame  EnableTorqueX=off  EnableTorqueY=off  EnableTorqueZ=off  EnableTorque=off  BlockFunction=simmechanics.library.forces_torques.external_force_torque
  PS Constant : fl_lib/Physical Signals/Sources/PS Constant  constant=1
  PS Constant1 : fl_lib/Physical Signals/Sources/PS Constant  constant=2*pi*L
  PS Constant2 : fl_lib/Physical Signals/Sources/PS Constant  constant=P
  PS Divide : fl_lib/Physical Signals/Functions/PS Divide
  PS Gain1 : fl_lib/Physical Signals/Functions/PS Gain  gain=1
  PS Product : fl_lib/Physical Signals/Functions/PS Product
  PS Product1 : fl_lib/Physical Signals/Functions/PS Product
  PS Saturation : fl_lib/Physical Signals/Nonlinear Operators/PS Saturation  Commented=on  upper_limit=-0.01  lower_limit=-inf
  PS Subtract : fl_lib/Physical Signals/Functions/PS Subtract
  PS-Simulink Converter : nesl_utility/PS-Simulink Converter  PhysicalDomain=network_engine_domain  SubClassName=ps_output  LeftPortType=input  RightPortType=output  PseudoPeriodic=off  Frequencies=[]  Unit=1  AffineConversion=off
  Pitch1 : fl_lib/Physical Signals/Functions/PS Gain  gain=kt*rho*Ap*Rp*Rp
  Pitch2 : fl_lib/Physical Signals/Functions/PS Gain  gain=-50
  Omega_x_body : PMIOPort  Port=1  Side=Left
  AlphaProp : PMIOPort  Port=2  Side=Left
  Thrust : PMIOPort  Port=3  Side=Right
  Prop Speed : PMIOPort  Port=4  Side=Right
  wires:
  PS-Simulink Converter/1 -> Display/1
  connections:
  PS Subtract/RConn1 -- PS Divide/LConn1
  PS Constant2/RConn1 -- PS Divide/LConn2
  PS-Simulink Converter/LConn1 -- PS Gain1/RConn1 -- PS Product1/LConn2
  PS Constant1/RConn1 -- PS Product/LConn1
  PS Product/LConn2 -- Omega_x_body/RConn1
  Pitch1/LConn1 -- PS Divide/RConn1
  PS Product1/LConn1 -- Pitch1/RConn1
  Pitch2/LConn1 -- PS Product1/RConn1
  PS Subtract/LConn2 -- PS Product/RConn1
  PS Subtract/LConn1 -- PS Constant/RConn1
  PS Gain1/LConn1 -- AlphaProp/RConn1
  External Force  and Torque1/RConn1 -- Thrust/RConn1
  External Force  and Torque1/LConn1 -- Prop Speed/RConn1 -- Pitch2/RConn1

== system QuadRotorPlant/External Force/Rotor2 ==
  Display : Display
  External Force  and Torque2 : sm_lib/Forces and Torques/External Force and Torque  ForceResolutionFrame=AttachedFrame  EnableForceX=off  EnableForceY=off  EnableForceZ=on  EnableForce=off  TorqueResolutionFrame=AttachedFrame  EnableTorqueX=off  EnableTorqueY=off  EnableTorqueZ=off  EnableTorque=off  BlockFunction=simmechanics.library.forces_torques.external_force_torque
  PS Constant : fl_lib/Physical Signals/Sources/PS Constant  constant=1
  PS Constant1 : fl_lib/Physical Signals/Sources/PS Constant  constant=-2*pi*L
  PS Constant2 : fl_lib/Physical Signals/Sources/PS Constant  constant=P
  PS Divide : fl_lib/Physical Signals/Functions/PS Divide
  PS Gain1 : fl_lib/Physical Signals/Functions/PS Gain  gain=1
  PS Product : fl_lib/Physical Signals/Functions/PS Product
  PS Product1 : fl_lib/Physical Signals/Functions/PS Product
  PS Saturation : fl_lib/Physical Signals/Nonlinear Operators/PS Saturation  Commented=on  upper_limit=inf  lower_limit=0.01
  PS Subtract : fl_lib/Physical Signals/Functions/PS Subtract
  PS-Simulink Converter : nesl_utility/PS-Simulink Converter  PhysicalDomain=network_engine_domain  SubClassName=ps_output  LeftPortType=input  RightPortType=output  PseudoPeriodic=off  Frequencies=[]  Unit=1  AffineConversion=off
  Pitch1 : fl_lib/Physical Signals/Functions/PS Gain  gain=kt*rho*Ap*Rp*Rp
  Pitch2 : fl_lib/Physical Signals/Functions/PS Gain  gain=50
  Omega_x_body : PMIOPort  Port=1  Side=Left
  AlphaProp : PMIOPort  Port=2  Side=Left
  Thrust1 : PMIOPort  Port=3  Side=Right
  Prop Speed : PMIOPort  Port=4  Side=Right
  wires:
  PS-Simulink Converter/1 -> Display/1
  connections:
  PS Subtract/RConn1 -- PS Divide/LConn1
  PS Constant2/RConn1 -- PS Divide/LConn2
  PS-Simulink Converter/LConn1 -- PS Product1/LConn2 -- PS Gain1/RConn1
  PS Constant1/RConn1 -- PS Product/LConn1
  PS Product/LConn2 -- Omega_x_body/RConn1
  Pitch1/LConn1 -- PS Divide/RConn1
  PS Product1/LConn1 -- Pitch1/RConn1
  Pitch2/LConn1 -- PS Product1/RConn1
  PS Subtract/LConn2 -- PS Product/RConn1
  PS Subtract/LConn1 -- PS Constant/RConn1
  PS Gain1/LConn1 -- AlphaProp/RConn1
  External Force  and Torque2/LConn1 -- Prop Speed/RConn1 -- Pitch2/RConn1
  External Force  and Torque2/RConn1 -- Thrust1/RConn1

== system QuadRotorPlant/External Force/Rotor3 ==
  Display : Display
  External Force  and Torque3 : sm_lib/Forces and Torques/External Force and Torque  ForceResolutionFrame=AttachedFrame  EnableForceX=off  EnableForceY=off  EnableForceZ=on  EnableForce=off  TorqueResolutionFrame=AttachedFrame  EnableTorqueX=off  EnableTorqueY=off  EnableTorqueZ=off  EnableTorque=off  BlockFunction=simmechanics.library.forces_torques.external_force_torque
  PS Constant : fl_lib/Physical Signals/Sources/PS Constant  constant=1
  PS Constant1 : fl_lib/Physical Signals/Sources/PS Constant  constant=-2*pi*L
  PS Constant2 : fl_lib/Physical Signals/Sources/PS Constant  constant=P
  PS Divide : fl_lib/Physical Signals/Functions/PS Divide
  PS Gain1 : fl_lib/Physical Signals/Functions/PS Gain  gain=1
  PS Product : fl_lib/Physical Signals/Functions/PS Product
  PS Product1 : fl_lib/Physical Signals/Functions/PS Product
  PS Saturation : fl_lib/Physical Signals/Nonlinear Operators/PS Saturation  Commented=on  upper_limit=inf  lower_limit=0.01
  PS Subtract : fl_lib/Physical Signals/Functions/PS Subtract
  PS-Simulink Converter : nesl_utility/PS-Simulink Converter  PhysicalDomain=network_engine_domain  SubClassName=ps_output  LeftPortType=input  RightPortType=output  PseudoPeriodic=off  Frequencies=[]  Unit=1  AffineConversion=off
  Pitch1 : fl_lib/Physical Signals/Functions/PS Gain  gain=kt*rho*Ap*Rp*Rp
  Pitch3 : fl_lib/Physical Signals/Functions/PS Gain  gain=50
  Omega_x_body : PMIOPort  Port=1  Side=Left
  AlphaProp : PMIOPort  Port=2  Side=Left
  Thrust : PMIOPort  Port=3  Side=Right
  Prop Speed : PMIOPort  Port=4  Side=Right
  wires:
  PS-Simulink Converter/1 -> Display/1
  connections:
  PS Subtract/RConn1 -- PS Divide/LConn1
  PS Constant2/RConn1 -- PS Divide/LConn2
  PS-Simulink Converter/LConn1 -- PS Gain1/RConn1 -- PS Product1/LConn2
  PS Constant1/RConn1 -- PS Product/LConn1
  PS Product/LConn2 -- Omega_x_body/RConn1
  Pitch1/LConn1 -- PS Divide/RConn1
  PS Product1/LConn1 -- Pitch1/RConn1
  Pitch3/LConn1 -- PS Product1/RConn1
  PS Subtract/LConn2 -- PS Product/RConn1
  PS Subtract/LConn1 -- PS Constant/RConn1
  PS Gain1/LConn1 -- AlphaProp/RConn1
  External Force  and Torque3/RConn1 -- Thrust/RConn1
  Pitch3/RConn1 -- Prop Speed/RConn1 -- External Force  and Torque3/LConn1

== system QuadRotorPlant/External Force/Rotor4 ==
  Display : Display
  External Force  and Torque4 : sm_lib/Forces and Torques/External Force and Torque  ForceResolutionFrame=AttachedFrame  EnableForceX=off  EnableForceY=off  EnableForceZ=on  EnableForce=off  TorqueResolutionFrame=AttachedFrame  EnableTorqueX=off  EnableTorqueY=off  EnableTorqueZ=off  EnableTorque=off  BlockFunction=simmechanics.library.forces_torques.external_force_torque
  PS Constant : fl_lib/Physical Signals/Sources/PS Constant  constant=1
  PS Constant1 : fl_lib/Physical Signals/Sources/PS Constant  constant=2*pi*L
  PS Constant2 : fl_lib/Physical Signals/Sources/PS Constant  constant=P
  PS Divide : fl_lib/Physical Signals/Functions/PS Divide
  PS Gain1 : fl_lib/Physical Signals/Functions/PS Gain  gain=1
  PS Product : fl_lib/Physical Signals/Functions/PS Product
  PS Product1 : fl_lib/Physical Signals/Functions/PS Product
  PS Saturation : fl_lib/Physical Signals/Nonlinear Operators/PS Saturation  Commented=on  upper_limit=-0.01  lower_limit=-inf
  PS Subtract : fl_lib/Physical Signals/Functions/PS Subtract
  PS-Simulink Converter : nesl_utility/PS-Simulink Converter  PhysicalDomain=network_engine_domain  SubClassName=ps_output  LeftPortType=input  RightPortType=output  PseudoPeriodic=off  Frequencies=[]  Unit=1  AffineConversion=off
  Pitch1 : fl_lib/Physical Signals/Functions/PS Gain  gain=kt*rho*Ap*Rp*Rp
  Pitch4 : fl_lib/Physical Signals/Functions/PS Gain  gain=-50
  Omega_x_body : PMIOPort  Port=1  Side=Left
  AlphaProp : PMIOPort  Port=2  Side=Left
  Thrust : PMIOPort  Port=3  Side=Right
  Prop Speed : PMIOPort  Port=4  Side=Right
  wires:
  PS-Simulink Converter/1 -> Display/1
  connections:
  PS Subtract/LConn1 -- PS Constant/RConn1
  PS Subtract/LConn2 -- PS Product/RConn1
  Pitch4/LConn1 -- PS Product1/RConn1
  PS Product1/LConn1 -- Pitch1/RConn1
  Pitch1/LConn1 -- PS Divide/RConn1
  PS Product/LConn2 -- Omega_x_body/RConn1
  PS Constant1/RConn1 -- PS Product/LConn1
  PS-Simulink Converter/LConn1 -- PS Gain1/RConn1 -- PS Product1/LConn2
  PS Constant2/RConn1 -- PS Divide/LConn2
  PS Subtract/RConn1 -- PS Divide/LConn1
  PS Gain1/LConn1 -- AlphaProp/RConn1
  Prop Speed/RConn1 -- External Force  and Torque4/LConn1 -- Pitch4/RConn1
  Thrust/RConn1 -- External Force  and Torque4/RConn1

== system QuadRotorPlant/Ground Stop/FloorStop1 ==
  6-DOF Joint1 : sm_lib/Joints/6-DOF Joint  SenseConstraintForce=off  SenseConstraintForceX=off  SenseConstraintForceY=off  SenseConstraintForceZ=off  SenseConstraintTorque=off  SenseConstraintTorqueX=off  SenseConstraintTorqueY=off  SenseConstraintTorqueZ=off  SenseTotalForce=off  SenseTotalForceX=off  SenseTotalForceY=off  SenseTotalForceZ=off  SenseTotalTorque=off  SenseTotalTorqueX=off  SenseTotalTorqueY=off  SenseTotalTorqueZ=off  CompositeWrenchDir=FollowerOnBase  CompositeWrenchFrame=BaseFrame  PxEquilibriumPosition=0  PxEquilibriumPositionUnits=m  PxSpringStiffness=0  PxSpringStiffnessUnits=N/m  PxDampingCoefficient=0  PxDampingCoefficientUnits=N/(m/s)  PxTorqueActuationMode=NoTorque  PxMotionActuationMode=ComputedMotion  PxSensePosition=off  PxSenseVelocity=off  PxSenseAcceleration=off  PxSenseTorqueForce=off  PxPositionTargetValue=1  PxPositionTargetValueUnits=m  PxPositionTargetSpecify=off  PxPositionTargetPriority=High  PxVelocityTargetValue=1  PxVelocityTargetValueUnits=m/s  PxVelocityTargetSpecify=off  PxVelocityTargetPriority=High  PyEquilibriumPosition=0  PyEquilibriumPositionUnits=m  PySpringStiffness=0  PySpringStiffnessUnits=N/m  PyDampingCoefficient=0  PyDampingCoefficientUnits=N/(m/s)  PyTorqueActuationMode=NoTorque  PyMotionActuationMode=ComputedMotion  PySensePosition=off  PySenseVelocity=off  PySenseAcceleration=off  PySenseTorqueForce=off  PyPositionTargetValue=0  PyPositionTargetValueUnits=m  PyPositionTargetSpecify=off  PyPositionTargetPriority=High  PyVelocityTargetValue=0  PyVelocityTargetValueUnits=m/s  PyVelocityTargetSpecify=off  PyVelocityTargetPriority=High  PzEquilibriumPosition=0  PzEquilibriumPositionUnits=m  PzSpringStiffness=0  PzSpringStiffnessUnits=N/m  PzDampingCoefficient=0  PzDampingCoefficientUnits=N/(m/s)  PzTorqueActuationMode=InputTorque  PzMotionActuationMode=ComputedMotion  PzSensePosition=on  PzSenseVelocity=on  PzSenseAcceleration=off  PzSenseTorqueForce=off  PzPositionTargetValue=-0.1  PzPositionTargetValueUnits=m  PzPositionTargetSpecify=off  PzPositionTargetPriority=High  PzVelocityTargetValue=0  PzVelocityTargetValueUnits=m/s  PzVelocityTargetSpecify=off  PzVelocityTargetPriority=High  SphDefPosRotationMethod=None  SphDefPosRotationAngleUnits=deg  SphDefPosRotationStandardAxis=+Z  SphDefPosRotationAngle=0  SphDefPosRotationArbitraryAxis=[0 0 1]  SphDefPosFollAlignAxisA=+X  SphDefPosBaseAlignAxisA=+Y  SphDefPosFollAlignAxisB=+Y  SphDefPosBaseAlignAxisB=+Z  SphDefPosRotationMatrix=[1 0 0; 0 1 0; 0 0 1]  SphEqPosRotationMethod=None  SphEqPosRotationAngleUnits=deg  SphEqPosRotationStandardAxis=+Z  SphEqPosRotationAngle=0  SphEqPosRotationArbitraryAxis=[0 0 1]  SphEqPosFollAlignAxisA=+X  SphEqPosBaseAlignAxisA=+Y  SphEqPosFollAlignAxisB=+Y  SphEqPosBaseAlignAxisB=+Z  SphEqPosRotationMatrix=[1 0 0; 0 1 0; 0 0 1]  SphSpringStiffness=0  SphSpringStiffnessUnits=N*m/deg  SphDampingCoefficient=0  SphDampingCoefficientUnits=N*m/(deg/s)  SphActuateTorqueX=off  SphActuateTorqueY=off  SphActuateTorqueZ=off  SphActuateTorque=off  SphTorqueActuationMode=NoTorque  SphMotionActuationMode=ComputedMotion  SphActuationFrame=BaseFrame  SphSensePosition=off  SphSenseVelocityX=off  SphSenseVelocityY=off  SphSenseVelocityZ=off  SphSenseVelocity=off  SphSenseAccelerationX=off  SphSenseAccelerationY=off  SphSenseAccelerationZ=off  SphSenseAcceleration=off  SphSenseTorqueX=off  SphSenseTorqueY=off  SphSenseTorqueZ=off  SphSenseTorqueForce=off  SphSensingFrame=BaseFrame  SphPositionTargetRotationMethod=StandardAxis  SphPositionTargetRotationAngleUnits=deg  SphPositionTargetRotationStandardAxis=+X  SphPositionTargetRotationAngle=10  SphPositionTargetRotationArbitraryAxis=[0 0 1]  SphPositionTargetFollAlignAxisA=+X  SphPositionTargetBaseAlignAxisA=+Y  SphPositionTargetFollAlignAxisB=+Y  SphPositionTargetBaseAlignAxisB=+Z  SphPositionTargetRotationMatrix=[1 0 0; 0 1 0; 0 0 1]  SphPositionTargetSpecify=off  SphPositionTargetPriority=High  SphVelocityTargetValue=[0 100 0]  SphVelocityTargetValueUnits=deg/s  SphVelocityTargetSpecify=off  SphVelocityTargetPriority=High  SphVelocityTargetInFollowerFrame=on  BlockFunction=simmechanics.library.joints.sixdof_joint
  Mechanical Translational Reference1 : fl_lib/Mechanical/Translational Elements/Mechanical Translational Reference
  PS Gain3 : fl_lib/Physical Signals/Functions/PS Gain  gain=1
  PS Gain4 : fl_lib/Physical Signals/Functions/PS Gain  gain=1
  Translational Simscape Intf1 : Subsystem
  Translational Hard Stop1 : fl_lib/Mechanical/Translational Elements/Translational Hard Stop  upper_bnd=100 m  lower_bnd=-zInit([0 2*Length 0],-Yaw0,GPitch,GRoll) m  stiff_up=1e6 N/m  stiff_low=Spring N/m  D_up=1500 N/(m/s)  D_low=Damp N/(m/s)  v_specify=off  v_priority=High  v=0 m/s  f_specify=off  f_priority=High  f=0 N  x_specify=on  x_priority=High  x=-zInit([0 2*Length 0],Yaw0,Pitch0,Roll0)+Alt m
  Conn1 : PMIOPort  Port=1  Side=Right
  Conn2 : PMIOPort  Port=2  Side=Left
  connections:
  PS Gain4/RConn1 -- 6-DOF Joint1/LConn2
  Translational Simscape Intf1/RConn1 -- PS Gain4/LConn1
  PS Gain3/LConn1 -- 6-DOF Joint1/RConn3
  Translational Hard Stop1/LConn1 -- Translational Simscape Intf1/LConn2
  PS Gain3/RConn1 -- Translational Simscape Intf1/LConn1
  Conn2/RConn1 -- 6-DOF Joint1/LConn1
  Translational Simscape Intf1/RConn2 -- Mechanical Translational Reference1/LConn1 -- Translational Hard Stop1/RConn1
  6-DOF Joint1/RConn1 -- Conn1/RConn1
